simulink model "wPIDwithoutRAD"  (R2025b)
settings: Solver=VariableStepAuto  StartTime=0.0  StopTime=1296  RelTol=1e-3
libraries: slpidlib x1
settings Model: Creator=suyas  LastModifiedBy=suyas

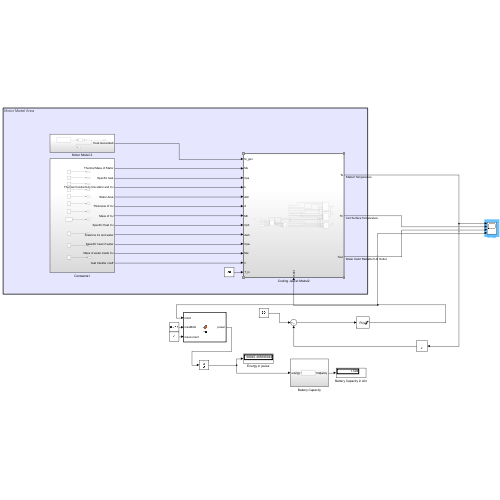
[thumbnail: Simulink's stored preview of the top-level diagram]
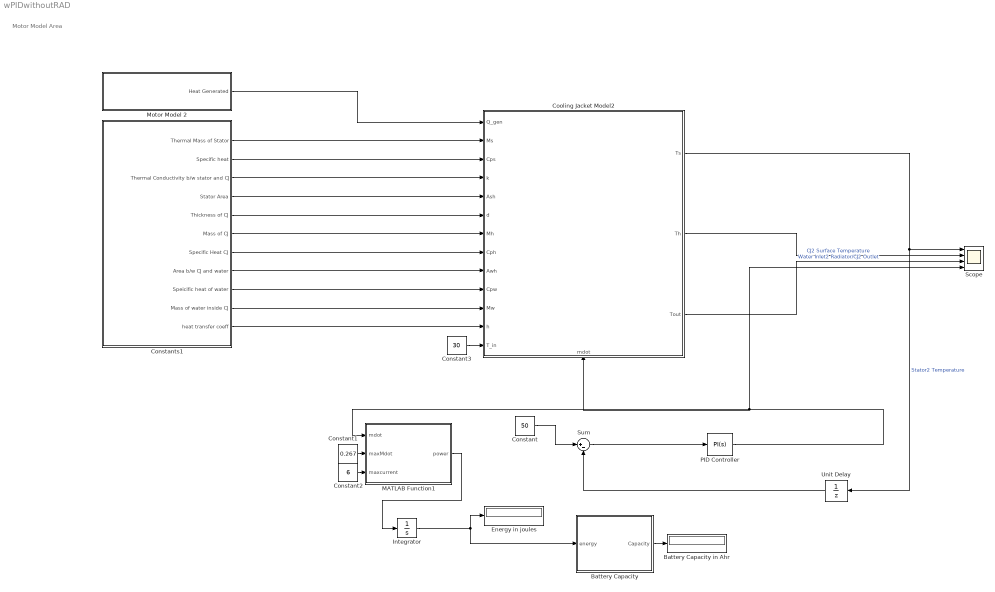
== system wPIDwithoutRAD ==
  note: Motor Model Area
  Battery Capacity : Subsystem
  Battery Capacity in Ahr : Display
  Constant : Constant  Value=50
  Constant1 : Constant  Value=0.267
  Constant2 : Constant  Value=6
  Constant3 : Constant  Value=30
  Constants1 : Subsystem
  Cooling Jacket Model2 : Subsystem
      settings: PortSchema="{\"entries\":[{\"content\":{\"sides\":[{\"content\":{\"connectorIds\":[\"In1\",\"In2\",\"In3\",\"In4\",\"In5\",\"In6\",\"In7\",\"In8\",\"In9\",\"In10\",\"In11\",\"In12\",\"In13\"]},\"type\":\"ConnectorPlacement.EquallySpacedRectSide\",\"uuid\":\"79d4d8e8-7803-45a2-afaa-4d22d6373157\"},{\"content\":{\"connectorIds\":[\"Out1\",\"Out2\",\"Out3\"],\"side\":\"RIGHT\"},\"type\":\"ConnectorPlacement.EquallySpacedRectSide\",\"uuid\":\"8eb2a985-3df9-4fca-ba99-d41949146ffd\"},{\"content\":{\"side\":\"TOP\"},\"type\":\"ConnectorPlacement.EquallySpacedRectSide\",\"uuid\":\"b6891a69-1971-4846-8973-0960fda02d22\"},{\"content\":{\"connectorIds\":[\"In14\"],\"side\":\"BOTTOM\"},\"type\":\"ConnectorPlacement.EquallySpacedRectSide\",\"uuid\":\"634c1221-39cf-4d03-a1b5-5507eb554710\"}]},\"type\":\"ConnectorPlacement.EquallySpacedConnector\",\"uuid\":\"d4f46766-14f9-4a8b-8c89-842668bdd4e0\"}],\"packageUris\":[\"http://schema.mathworks.com/mf0/Connector/R2020b\"],\"version\":\"1.0\"}"
  Energy in joules : Display
  Integrator : Integrator
  MATLAB Function1 : MATLAB Function  TreatAsAtomicUnit=on
  Motor Model 2 : Subsystem
  PID Controller : slpidlib/PID Controller  Controller=PI  Form=Parallel  TimeDomain=Continuous-time  UseExternalTs=off  SampleTime=-1  IntegratorMethod=Forward Euler  FilterMethod=Forward Euler  ControllerParametersSource=internal  P=-0.127089567461861  I=-0.0157501490032625  UseKiTs=off  D=0.224846252339156  UseExternalDerivativeSource=off  N=0.0268819532474394  UseFilter=on  TunerSelectOption=Transfer Function Based (PID Tuner App)  InitialConditionSource=internal  InitialConditionForIntegrator=0  InitialConditionForFilter=0  DifferentiatorICPrevScaledInput=0  ExternalReset=none  TrackingMode=off  Kt=1  LimitOutput=on  SatLimitsSource=internal  UpperSaturationLimit=0.267  LowerSaturationLimit=0  LinearizeAsGain=on  AntiWindupMode=back-calculation  Kb=1  LimitIntegrator=on  UpperIntegratorSaturationLimit=0.267  LowerIntegratorSaturationLimit=0  POutMin=[]  POutMax=[]  IOutMin=[]  IOutMax=[]  DOutMin=[]  DOutMax=[]  NOutMin=[]  NOutMax=[]  SumOutMin=[]  SumOutMax=[]  SaturationOutMin=[]  SaturationOutMax=[]  PParamMin=[]  PParamMax=[]  IParamMin=[]  IParamMax=[]  DParamMin=[]  DParamMax=[]  NParamMin=[]  NParamMax=[]  KbParamMin=[]  KbParamMax=[]  KtParamMin=[]  KtParamMax=[]  KbOutMin=[]  KbOutMax=[]  KtOutMin=[]  KtOutMax=[]  IntegratorOutMin=[]  IntegratorOutMax=[]  FilterOutMin=[]  FilterOutMax=[]  SumI1OutMin=[]  SumI1OutMax=[]  SumI2OutMin=[]  SumI2OutMax=[]  SumI3OutMin=[]  SumI3OutMax=[]  SumI4OutMin=[]  SumI4OutMax=[]  SumDOutMin=[]  SumDOutMax=[]  DifferentiatorOutMin=[]  DifferentiatorOutMax=[]  FilterDiffOutCoefMin=[]  FilterDiffOutCoefMax=[]  ReciprocalOutMin=[]  ReciprocalOutMax=[]  SumDenOutMin=[]  SumDenOutMax=[]  SumNumOutMin=[]  SumNumOutMax=[]  DivideOutMin=[]  DivideOutMax=[]  UdiffTsProdOutMin=[]  UdiffTsProdOutMax=[]  NTsProdOutMin=[]  NTsProdOutMax=[]  UintegralTsProdOutMin=[]  UintegralTsProdOutMax=[]  UngainTsProdOutMin=[]  UngainTsProdOutMax=[]  ClampingZeroOutDataTypeStr=Inherit: Inherit via back propagation  ClampingZeroOutMin=[]  ClampingZeroOutMax=[]  FilterDenConstantOutDataTypeStr=Inherit: Inherit via back propagation  FilterDenConstantOutMin=[]  FilterDenConstantOutMax=[]  PCopyOutDataTypeStr=Inherit: Inherit via back propagation  PCopyOutMin=[]  PCopyOutMax=[]  NCopyOutDataTypeStr=Inherit: Inherit via back propagation  NCopyOutMin=[]  NCopyOutMax=[]  IntegratorContinuousStateAttributes=''  IntegratorStateMustResolveToSignalObject=off  IntegratorRTWStateStorageClass=Auto  FilterContinuousStateAttributes=''  FilterStateMustResolveToSignalObject=off  FilterRTWStateStorageClass=Auto  ParallelPVariant=InternalParameters  IdealPVariant=Disabled  IVariant=InternalParameters  DVariant=Disabled  IntegratorVariant=Continuous  SatVariant=Enabled  AWVariant=BackCalculation  PCopyVariant=Disabled  TRVariant=Disabled  FdbkBlocksVariant=Forward  IdealPFdbkVariant=Disabled  SatFdbkVariant=Disabled  DerivativeFilterVariant=Disabled  NVariant=Disabled  NCopyVariant=Disabled_SignalSpec  FilterICVariant=Disabled  IntegratorICVariant=InternalICs  ExternalResetVariant=Disabled  TRSumVariant=Passthrough  SumFdbkVariant=Disabled  SumVariant=Sum_PI  TsampFilterVariant=InternalTs  TsampNgainVariant=Passthrough  TsampIntegralVariant=Disabled_SignalSpec  ExternalSaturationOutDataTypeStr=Inherit: Same as second input  DerivativeSourceVariant=Disabled  PreIntVariant=InternalPreInt
  Scope : Scope  NumInputPorts=4
      settings: ActiveDisplayYMinimum=47.723771460412486  ActiveDisplayYMaximum=52.2356856322447
  Sum : Sum  Inputs=|+-
  Unit Delay : UnitDelay  SampleTime=0.001  HasFrameUpgradeWarning=on
  wires:
  Constant/1 -> Sum/1
  Constant3/1 -> Cooling Jacket Model2/13(T_in)
  PID Controller/1 -> MATLAB Function1/1(mdot), Cooling Jacket Model2/14(mdot), Scope/4
  Constants1/8(Area b/w CJ and water) -> Cooling Jacket Model2/9(Awh)
  Constants1/5(Thickness of CJ) -> Cooling Jacket Model2/6(d)
  Constants1/9(Speicific heat of water) -> Cooling Jacket Model2/10(Cpw)
  Cooling Jacket Model2/2(Th) -> Scope/2  "CJ2 Surface Temperature"
  Constants1/6(Mass of CJ) -> Cooling Jacket Model2/7(Mh)
  Constants1/3(Thermal Conductivity b/w stator and CJ) -> Cooling Jacket Model2/4(k)
  Cooling Jacket Model2/1(Ts) -> Unit Delay/1, Scope/1  "Stator2 Temperature"
  Constants1/7(Specific Heat CJ) -> Cooling Jacket Model2/8(Cph)
  Cooling Jacket Model2/3(Tout) -> Scope/3  "Water Inlet2 Radiator/CJ2 Outlet"
  Constants1/10(Mass of water inside CJ) -> Cooling Jacket Model2/11(Mw)
  Constants1/4(Stator Area) -> Cooling Jacket Model2/5(Ash)
  Constants1/2(Specific heat) -> Cooling Jacket Model2/3(Cps)
  Constants1/11(heat transfer coeff) -> Cooling Jacket Model2/12(h)
  Sum/1 -> PID Controller/1
  Constants1/1(Thermal Mass of Stator) -> Cooling Jacket Model2/2(Ms)
  Unit Delay/1 -> Sum/2
  Motor Model 2/1(Heat Generated) -> Cooling Jacket Model2/1(Q_gen)
  Integrator/1 -> Battery Capacity/1(energy), Energy in joules/1
  Battery Capacity/1(Capacity) -> Battery Capacity in Ahr/1
  MATLAB Function1/1(power) -> Integrator/1
  Constant2/1 -> MATLAB Function1/3(maxcurrent)
  Constant1/1 -> MATLAB Function1/2(maxMdot)

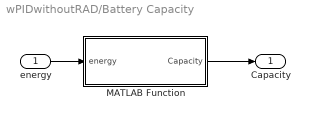
== system wPIDwithoutRAD/Battery Capacity ==
  energy : Inport
  MATLAB Function : MATLAB Function  TreatAsAtomicUnit=on
  Capacity : Outport
  wires:
  energy/1 -> MATLAB Function/1(energy)
  MATLAB Function/1(Capacity) -> Capacity/1

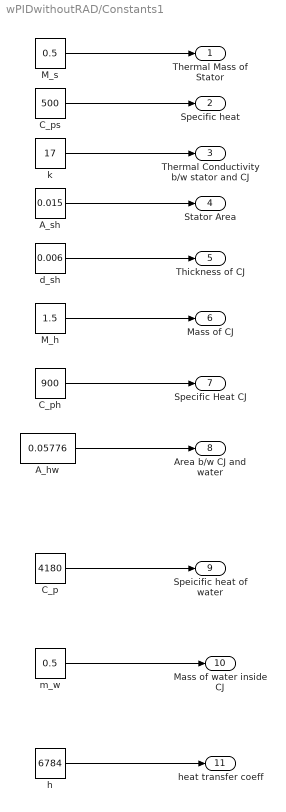
== system wPIDwithoutRAD/Constants1 ==
  A_hw : Constant  Value=0.05776
  A_sh : Constant  Value=0.015
  C_p : Constant  Value=4180
  C_ph : Constant  Value=900
  C_ps : Constant  Value=500
  M_h : Constant  Value=1.5
  M_s : Constant  Value=0.5
  d_sh : Constant  Value=0.006
  h : Constant  Value=6784
  k : Constant  Value=17
  m_w : Constant  Value=0.5
  Thermal Mass of Stator : Outport
  Specific heat : Outport  Port=2
  Thermal Conductivity b/w stator and CJ : Outport  Port=3
  Stator Area : Outport  Port=4
  Thickness of CJ : Outport  Port=5
  Mass of CJ : Outport  Port=6
  Specific Heat CJ : Outport  Port=7
  Area b/w CJ and water : Outport  Port=8
  Speicific heat of water : Outport  Port=9
  Mass of water inside CJ : Outport  Port=10
  heat transfer coeff : Outport  Port=11
  wires:
  C_ph/1 -> Specific Heat CJ/1
  A_sh/1 -> Stator Area/1
  C_ps/1 -> Specific heat/1
  M_s/1 -> Thermal Mass of Stator/1
  d_sh/1 -> Thickness of CJ/1
  m_w/1 -> Mass of water inside CJ/1
  k/1 -> Thermal Conductivity b/w stator and CJ/1
  M_h/1 -> Mass of CJ/1
  A_hw/1 -> Area b/w CJ and water/1
  C_p/1 -> Speicific heat of water/1
  h/1 -> heat transfer coeff/1

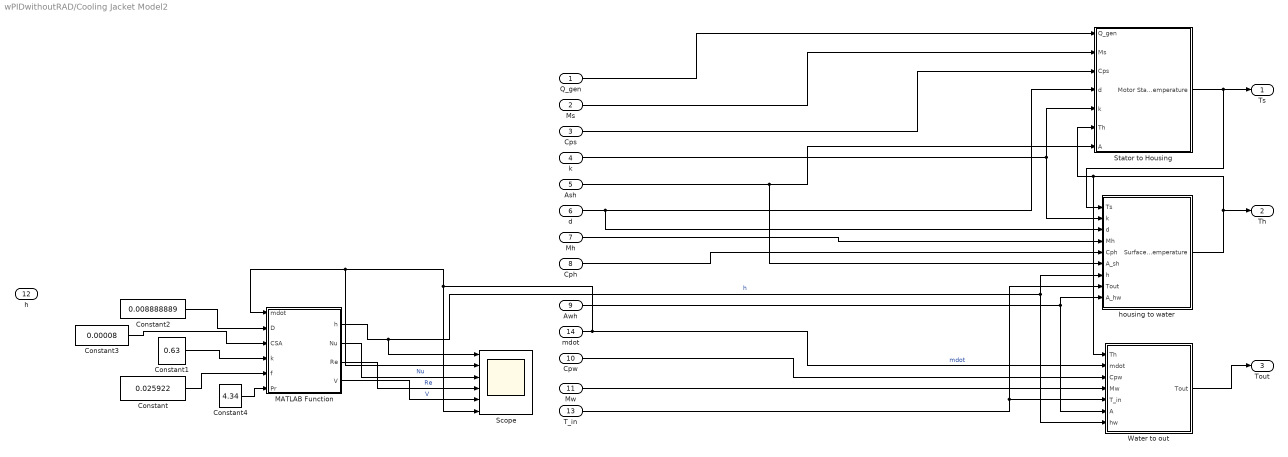
== system wPIDwithoutRAD/Cooling Jacket Model2 ==
  Q_gen : Inport
  Ms : Inport  Port=2
  Cps : Inport  Port=3
  k : Inport  Port=4
  Ash : Inport  Port=5
  d : Inport  Port=6
  Mh : Inport  Port=7
  Cph : Inport  Port=8
  Awh : Inport  Port=9
  Cpw : Inport  Port=10
  Mw : Inport  Port=11
  h : Inport  Port=12
  T_in : Inport  Port=13
  mdot : Inport  Port=14
  Constant : Constant  Value=0.025922
  Constant1 : Constant  Value=0.63
  Constant2 : Constant  Value=0.008888889
  Constant3 : Constant  Value=0.00008
  Constant4 : Constant  Value=4.34
  MATLAB Function : MATLAB Function  TreatAsAtomicUnit=on
  Scope : Scope  NumInputPorts=6
      settings: ActiveDisplayYMinimum=-1  ActiveDisplayYMaximum=1
  Stator to Housing : Subsystem
  Water to out : Subsystem
  housing to water : Subsystem
  Ts : Outport
  Th : Outport  Port=2
  Tout : Outport  Port=3
  wires:
  mdot/1 -> Scope/2, MATLAB Function/1(mdot), Scope/6, Water to out/2(mdot)  "mdot"
  Stator to Housing/1(Motor Stator Temperature) -> Ts/1, housing to water/1(Ts)
  Water to out/1(Tout) -> Tout/1
  housing to water/1(Surface Temperature) -> Stator to Housing/6(Th), Water to out/1(Th), Th/1
  d/1 -> housing to water/3(d), Stator to Housing/4(d)
  Cpw/1 -> Water to out/3(Cpw)
  Mw/1 -> Water to out/4(Mw)
  Q_gen/1 -> Stator to Housing/1(Q_gen)
  Ms/1 -> Stator to Housing/2(Ms)
  Cps/1 -> Stator to Housing/3(Cps)
  Ash/1 -> housing to water/6(A_sh), Stator to Housing/7(A)
  T_in/1 -> housing to water/8(Tout), Water to out/5(T_in)
  Mh/1 -> housing to water/4(Mh)
  Cph/1 -> housing to water/5(Cph)
  k/1 -> housing to water/2(k), Stator to Housing/5(k)
  MATLAB Function/1(h) -> Scope/1, housing to water/7(h), Water to out/7(hw)  "h"
  Awh/1 -> housing to water/9(A_hw), Water to out/6(A)
  Constant/1 -> MATLAB Function/5(f)
  Constant1/1 -> MATLAB Function/4(k)
  Constant2/1 -> MATLAB Function/2(D)
  Constant3/1 -> MATLAB Function/3(CSA)
  Constant4/1 -> MATLAB Function/6(Pr)
  MATLAB Function/2(Nu) -> Scope/3  "Nu"
  MATLAB Function/3(Re) -> Scope/4  "Re"
  MATLAB Function/4(V) -> Scope/5  "V"

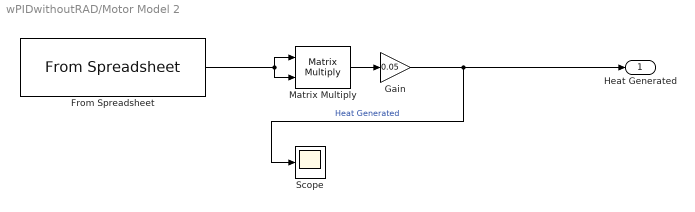
== system wPIDwithoutRAD/Motor Model 2 ==
  From Spreadsheet : FromSpreadsheet  FileName=C:\Users\suyas\Desktop\CurrentvTime (2).xlsx
  Gain : Gain  Gain=0.05
  Matrix Multiply : Product  Multiplication=Matrix(*)
  Scope : Scope
      settings: ActiveDisplayYMinimum=-88.25227  ActiveDisplayYMaximum=794.27044  DataLoggingVariableName=ScopeData2
  Heat Generated : Outport
  wires:
  Matrix Multiply/1 -> Gain/1
  From Spreadsheet/1 -> Matrix Multiply/2, Matrix Multiply/1
  Gain/1 -> Scope/1, Heat Generated/1  "Heat Generated"

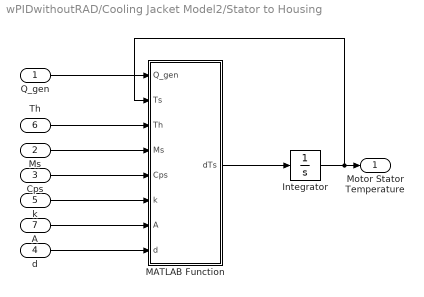
== system wPIDwithoutRAD/Cooling Jacket Model2/Stator to Housing ==
  Q_gen : Inport
  Ms : Inport  Port=2
  Cps : Inport  Port=3
  d : Inport  Port=4
  k : Inport  Port=5
  Th : Inport  Port=6
  A : Inport  Port=7
  Integrator : Integrator  InitialCondition=35
  MATLAB Function : MATLAB Function  TreatAsAtomicUnit=on
  Motor Stator Temperature : Outport
  wires:
  MATLAB Function/1(dTs) -> Integrator/1
  Cps/1 -> MATLAB Function/5(Cps)
  k/1 -> MATLAB Function/6(k)
  Ms/1 -> MATLAB Function/4(Ms)
  d/1 -> MATLAB Function/8(d)
  A/1 -> MATLAB Function/7(A)
  Q_gen/1 -> MATLAB Function/1(Q_gen)
  Integrator/1 -> MATLAB Function/2(Ts), Motor Stator Temperature/1
  Th/1 -> MATLAB Function/3(Th)

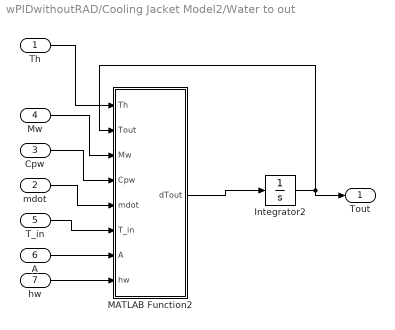
== system wPIDwithoutRAD/Cooling Jacket Model2/Water to out ==
  Th : Inport
  mdot : Inport  Port=2
  Cpw : Inport  Port=3
  Mw : Inport  Port=4
  T_in : Inport  Port=5
  A : Inport  Port=6
  hw : Inport  Port=7
  Integrator2 : Integrator  InitialCondition=35
  MATLAB Function2 : MATLAB Function  TreatAsAtomicUnit=on
  Tout : Outport
  wires:
  Integrator2/1 -> Tout/1, MATLAB Function2/2(Tout)
  MATLAB Function2/1(dTout) -> Integrator2/1
  Th/1 -> MATLAB Function2/1(Th)
  T_in/1 -> MATLAB Function2/6(T_in)
  Mw/1 -> MATLAB Function2/3(Mw)
  mdot/1 -> MATLAB Function2/5(mdot)
  Cpw/1 -> MATLAB Function2/4(Cpw)
  A/1 -> MATLAB Function2/7(A)
  hw/1 -> MATLAB Function2/8(hw)

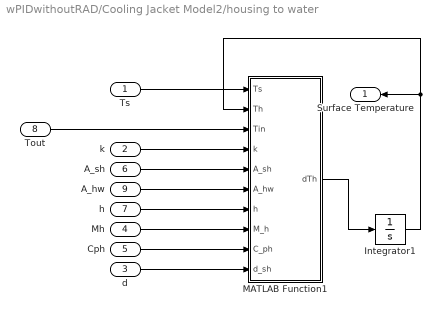
== system wPIDwithoutRAD/Cooling Jacket Model2/housing to water ==
  Ts : Inport
  k : Inport  Port=2
  d : Inport  Port=3
  Mh : Inport  Port=4
  Cph : Inport  Port=5
  A_sh : Inport  Port=6
  h : Inport  Port=7
  Tout : Inport  Port=8
  A_hw : Inport  Port=9
  Integrator1 : Integrator  InitialCondition=35
  MATLAB Function1 : MATLAB Function  TreatAsAtomicUnit=on
  Surface Temperature : Outport
  wires:
  MATLAB Function1/1(dTh) -> Integrator1/1
  k/1 -> MATLAB Function1/4(k)
  Ts/1 -> MATLAB Function1/1(Ts)
  Tout/1 -> MATLAB Function1/3(Tin)
  Integrator1/1 -> MATLAB Function1/2(Th), Surface Temperature/1
  d/1 -> MATLAB Function1/10(d_sh)
  Cph/1 -> MATLAB Function1/9(C_ph)
  Mh/1 -> MATLAB Function1/8(M_h)
  A_hw/1 -> MATLAB Function1/6(A_hw)
  A_sh/1 -> MATLAB Function1/5(A_sh)
  h/1 -> MATLAB Function1/7(h)

== matlab function wPIDwithoutRAD/MATLAB Function1 ==
  data: mdot input; power output; maxMdot input; maxcurrent input
function power = fcn(mdot, maxMdot, maxcurrent)
    power = (((4-maxcurrent)/(0-maxMdot))*(mdot - maxMdot) + maxcurrent)*12;
end

== matlab function wPIDwithoutRAD/Cooling Jacket Model2/MATLAB Function ==
  data: mdot input; h output; D input; CSA input; k input; f input; Pr input; Nu output; Re output; V output
function [h, Nu, Re, V]= fcn(mdot, D, CSA, k, f, Pr)
V = mdot/(1000*CSA);
Re = (V*1000*D)/0.00089;
Nu = ((f/8)*(Re-1000)*Pr)/(1+(12.7*(f/8)^0.5 * (Pr^(2/3) - 1)));
h = (Nu*k)/D;
end

== matlab function wPIDwithoutRAD/Battery Capacity/MATLAB Function ==
  data: Capacity output; energy input
function Capacity = fcn(energy)
    Capacity = energy/(12*3600);
end

== matlab function wPIDwithoutRAD/Cooling Jacket Model2/Stator to Housing/MATLAB Function ==
  data: Q_gen input; Ts input; dTs output; Th input; Ms input; Cps input; k input; A input; d input
function dTs = f1(Q_gen, Ts, Th, Ms, Cps, k, A, d)
    dTs = (Q_gen - (Ts - Th) * k * A / d) / (Ms * Cps);
end

== matlab function wPIDwithoutRAD/Cooling Jacket Model2/Water to out/MATLAB Function2 ==
  data: Th input; Tout input; Mw input; Cpw input; mdot input; T_in input; dTout output; A input; hw input
function dTout = f3(Th, Tout, Mw, Cpw, mdot, T_in, A, hw)
    q_from_housing = (Th - Tout) * hw * A;
    q_out = (Tout - T_in) * mdot * Cpw;
    dTout = (q_from_housing - q_out) / (Mw * Cpw);
end

== matlab function wPIDwithoutRAD/Cooling Jacket Model2/housing to water/MATLAB Function1 ==
  data: Ts input; Th input; Tin input; k input; A_sh input; A_hw input; dTh output; h input; M_h input; C_ph input; d_sh input
function dTh = f2(Ts, Th, Tin, k, A_sh, A_hw, h, M_h, C_ph, d_sh)
    dTh = ((k*A_sh*(Ts - Th)/d_sh) - h*A_hw*(Th - Tin)) / (M_h * C_ph);
end
